simulink model "fit6DoF_th"  (R2018b)
settings: Solver=VariableStepAuto  StartTime=0.0  StopTime=0  RelTol=1e-3
values from neighbouring files (symbols this model uses):
  R = [r1(:) r2(:) r3(:) r4(:)]    [perfIndx_ts1.m]
  U = [u1(:) u2(:) u3(:) u4(:)]    [perfIndx_ts1.m]
  w = ones([1 numDots])    [fit6DoFDoF_ts1.m]    (also in perfIndx_ts1.m = [1 1 1 1])
undefined symbols (not defined in the file or in its folder): DBdyTrue
libraries: fit6DoF x1
settings Model: SimulationMode=rapid-accelerator  Creator=M.Cobb  LastModifiedBy=M.Cobb

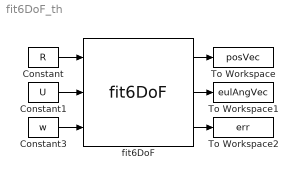
== system fit6DoF_th ==
  Constant : Constant  Value=R
  Constant1 : Constant  Value=U
  Constant3 : Constant  Value=w
  To Workspace : ToWorkspace  VariableName=posVec  SaveFormat=Structure With Time  SampleTime=-1
  To Workspace1 : ToWorkspace  VariableName=eulAngVec  SaveFormat=Structure With Time  SampleTime=-1
  To Workspace2 : ToWorkspace  VariableName=err  SaveFormat=Structure With Time  SampleTime=-1
  fit6DoF : fit6DoF/fit6DoF  D=DBdyTrue  initPosVec=[0 0 50]  initEulAng=[0 0 0]*pi/180  HInvInit=eye(6)  maxIBFGS=1000  posTolBFGS=0.05  angTolBFGS=0.05*pi/180  dxPos=0.0001*[1 1 1]  dxEul=0.01*[1 1 1]*pi/180  stepSize=1e-4  maxIBP=1000  maxIGS=1000  posTolGS=0.05  angTolGS=0.05*pi/180
  wires:
  fit6DoF/1 -> To Workspace/1
  fit6DoF/2 -> To Workspace1/1
  fit6DoF/3 -> To Workspace2/1
  Constant/1 -> fit6DoF/1
  Constant1/1 -> fit6DoF/2
  Constant3/1 -> fit6DoF/3
